simulink model "gr_onda"  (R2022b)
settings: Solver=ode45  StartTime=0.0  StopTime=1.5  RelTol=1e-3
settings Model: Creator=FELIPE OCAMPO  LastModifiedBy=Catalina

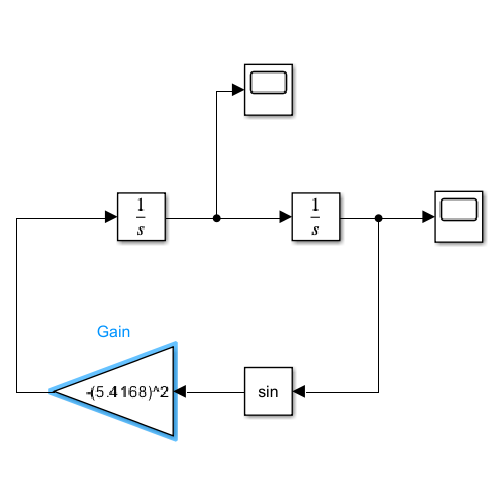
[thumbnail: Simulink's stored preview of the top-level diagram]
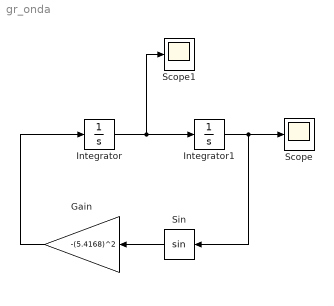
== system gr_onda ==
  Gain : Gain  Gain=-(5.4168)^2
  Integrator : Integrator
  Integrator1 : Integrator  InitialCondition=0.8116
  Scope : Scope
  Scope1 : Scope
  Sin : Trigonometry
  wires:
  Integrator/1 -> Scope1/1, Integrator1/1
  Gain/1 -> Integrator/1
  Integrator1/1 -> Scope/1, Sin/1
  Sin/1 -> Gain/1
